simulink model "F16ASYM_Controlled"  (R2015a)
settings: Solver=ode3  SolverMode=SingleTasking  StartTime=0.0  StopTime=inf  FixedStep=T_sim  RelTol=1e-3
InitFcn:
  | load('NN_c_weights_Last_stable.mat')
StopFcn:
  | Final_results
values from neighbouring files (symbols this model uses):
  a1 = fitresult.p1    [Stall_protection.m]
  alpha_map_eval = ones(size(M_eval))*NaN    [Auto_trim_aid.m]    (also in Autotrim_maps.mat = [nan nan 0.277598136245 0.119432432992 0.0579479097061 0.027)
  beta_map_eval = ones(size(M_eval))*NaN    [Auto_trim_aid.m]    (also in Autotrim_maps.mat = [nan nan -0.00151549403324 0.00117807579006 -0.0052086799721)
  C_L_0 = fitresult.p2    [Stall_protection.m]
  G_eval = NaN*ones(size(M_sq,2),size(H_sq,2))    [Stall_protection.m]
  H_sq = unique(sort(H_sq))    [Stall_protection.m]
  H_sq_autotrim = min( F_envelope.H_1g):2000:max(F_envelope.H_1g)    [Auto_trim_aid.m]    (also in Autotrim_maps.mat = [0 2000 4000 6000 8000 10000 12000 14000 16000 18000])
  K_b_q_extrap_ACC = K_b_q_extrap    [RUN_ME.m]
  K_b_q_extrap_AoA = K_b_q_extrap    [RUN_ME.m]
  M_sq = unique(sort(M_sq))    [Stall_protection.m]
  M_sq_autotrim = 0:0.1:max(F_envelope.M_1g)    [Auto_trim_aid.m]    (also in Autotrim_maps.mat = [0 0.1 0.2 0.3 0.4 0.5 0.6 0.7 0.8 0.9 1 1.1 ... (21 element)
  T_sim = 0.02    [RUN_ME.m]
  tau_q_extrap_ACC = tau_q_extrap    [RUN_ME.m]
  tau_q_extrap_AoA = tau_q_extrap    [RUN_ME.m]
  velocity = M_eval(I,J)*a    [Auto_trim_aid.m]
undefined symbols (not defined in the file or in its folder): ACCEL, B, Earth, fi_flag_Simulink, GYRO, H_sq_sche, k_B, K_b_ACC_extrap, K_b_AoA_extrap, latitude, longitude, m, m_B, M_sq_sche, Model_used_flag, rad, s, sigbuilder_block, Stall_curve, tau_ACC_extrap, tau_AoA_extrap, Theta_1_roll_last, Theta_2_roll_last, Theta_3_roll_last, trim_control, trim_state, trim_throttle, V_Comp_A_w_z_last, V_Comp_last, V_Comp_last_ONE, V_long_lastA_w_z, V_long_lastAoA, V_roll_last, V_roll_lastMOD, V_yaw_last, W_Comp_A_w_z_last, W_Comp_last, W_long_lastA_w_z, W_long_lastAoA, W_roll_last, W_roll_lastMOD, W_yaw_last, WGS84
libraries: Adaptive_FaultTolerantControl x57, dspsigops x37, F16_Actuator_Library x14, commnoisgen2 x13, simulink x11, simulink_extras x10, dsparch4 x6, aerolibatmos2 x6, aerolibtransform2 x6, aerolibfltsims x3, dspvision x3, dspsnks4 x3
(part 12 of 14)

== system F16ASYM_Controlled/Primary Controller/P controller + adaptive Isolated NN/On-line (adaptive) multi-layer NNs SIMPL/Roll NN/Roll 2HL NN ==
  note: Be careful with dimensions of inputs!!!
      | NORMALIZATION!!!
  v_ad^ prev : Inport
  p_chanel vars : Inport  Port=2
  All_meas : Inport  Port=3
  Roll_learning rate : Inport  Port=4
  Roll reg param : Inport  Port=5
  " " : ToWorkspace  VariableName=Theta_3_roll_last  SampleTime=-1
      settings: MaxDataPoints=1
  "  " : Memory  X0=Theta_3_roll_last
  "   " : Memory  X0=Theta_2_roll_last
  B : Constant
  Bus Selector1 : BusSelector  OutputSignals=p_err,p_sf,p_sf_dot,K_b_p
  Bus Selector2 : BusSelector  OutputSignals=signal1.Alt meas (m),signal2.Mach,signal1.AoA meas (rad),signal1.SS meas (rad),signal1.omega_b meas (rad/s)
  Constant : Constant
  Constant2 : Constant
  Display : Display
  Divide : Product  Inputs=**
  Divide1 : Product  Inputs=**
  Divide2 : Product  Inputs=*/
  Gain : Gain  Gain=1/15000
  Memory2 : Memory  X0=Theta_1_roll_last
  Mux : Mux  Inputs=12
  Roll Multilayer NN : MATLAB Function  TreatAsAtomicUnit=on
  Scope : Scope
      settings: YMin=-14  YMax=4  SaveName=ScopeData16
  Selector : Selector  InputPortWidth=3  Indices=3
  Terminator : Terminator
  Terminator1 : Terminator
  To Workspace : ToWorkspace  VariableName=Theta_1_roll_last  SampleTime=-1
      settings: MaxDataPoints=1
  To Workspace1 : ToWorkspace  VariableName=Theta_2_roll_last  SampleTime=-1
      settings: MaxDataPoints=1
  v_ad_comp : Outport
  wires:
  Roll Multilayer NN/3(Z_norm_unit) -> Terminator1/1
  Mux/1 -> Roll Multilayer NN/1(X_bar), Scope/1, Display/1
  Roll reg param/1 -> Roll Multilayer NN/6(Roll_reg_param)
  Roll_learning rate/1 -> Roll Multilayer NN/5(Roll_learnign_rate)
  Memory2/1 -> Roll Multilayer NN/7(Theta_1)
  Roll Multilayer NN/5(Theta_2_update) -> "   "/1, To Workspace1/1
  "  "/1 -> Roll Multilayer NN/9(Theta_3)
  Roll Multilayer NN/6(Theta_3_update) -> " "/1, "  "/1
  Bus Selector2/2 -> Mux/3, Divide/1, Divide/2  "<Mach>"
  Constant2/1 -> Divide2/1
  Bus Selector1/4 -> Divide2/2  "<K_b_p>"
  Divide2/1 -> [P]
  Roll Multilayer NN/2(v_ad) -> Terminator/1
  Roll Multilayer NN/4(Theta_1_update) -> Memory2/1, To Workspace/1
  v_ad^ prev/1 -> Mux/12
  [P] -> Roll Multilayer NN/3(P)
  B/1 -> Roll Multilayer NN/4(B)
  "   "/1 -> Roll Multilayer NN/8(Theta_2)
  Roll Multilayer NN/1(v_ad_comp) -> v_ad_comp/1
  Selector/1 -> Mux/8
  Bus Selector2/5 -> Selector/1  "<omega_b meas (rad/s)>"
  Gain/1 -> Mux/2
  Bus Selector2/4 -> Mux/7  "<SS meas (rad)>"
  Divide1/1 -> Mux/6
  Bus Selector2/3 -> Mux/5, Divide1/1, Divide1/2  "<AoA meas (rad)>"
  Divide/1 -> Mux/4
  Bus Selector2/1 -> Gain/1  "<Alt meas (m)>"
  All_meas/1 -> Bus Selector2/1
  Constant/1 -> Mux/1
  Bus Selector1/1 -> Roll Multilayer NN/2(e), Mux/9  "<p_err>"
  Bus Selector1/3 -> Mux/11  "<p_sf_dot>"
  Bus Selector1/2 -> Mux/10  "<p_sf>"
  p_chanel vars/1 -> Bus Selector1/1

== system F16ASYM_Controlled/Primary Controller/P controller + adaptive Isolated NN/On-line (adaptive) multi-layer NNs SIMPL/Yaw Chanel/Yaw HL NN ==
  note: Be careful with dimensions of inputs!!!
      | NORMALIZATION!!!
  v_ad^ prev : Inport
  Yaw_chanel vars : Inport  Port=2
  All_meas : Inport  Port=3
  Yaw_learning rate : Inport  Port=4
  Yaw reg param : Inport  Port=5
  Bus Selector1 : BusSelector  OutputSignals=beta_chanel vars.beta_err,r_chanel vars.r_err,beta_chanel vars.beta_sf,beta_chanel vars.beta_sf_dot,r_chanel vars.r_sf_dot,beta_chanel vars.K_b_beta,r_chanel vars.K_b_r
  Bus Selector2 : BusSelector  OutputSignals=signal1.Alt meas (m),signal2.Mach,signal1.AoA meas (rad),signal1.Euler meas (rad)
  Constant : Constant
  Constant1 : Constant  Value=[0;1]
  Display : Display
  Divide : Product  Inputs=**
  Gain : Gain  Gain=1/15000
  Memory2 : Memory  X0=V_yaw_last
  Memory3 : Memory  X0=W_yaw_last
  Mux : Mux  Inputs=12
  Mux1 : Mux  Inputs=2
  Mux2 : Mux  Inputs=2
  Scope : Scope
      settings: YMin=-0.25  YMax=3.75  SaveName=ScopeData17
  Selector : Selector  InputPortWidth=3
  Terminator : Terminator
  Terminator1 : Terminator
  To Workspace : ToWorkspace  VariableName=V_yaw_last  SampleTime=-1
      settings: MaxDataPoints=1
  To Workspace1 : ToWorkspace  VariableName=W_yaw_last  SampleTime=-1
      settings: MaxDataPoints=1
  Yaw NN : MATLAB Function  TreatAsAtomicUnit=on
  v_ad_comp : Outport
  wires:
  Yaw NN/3(Z_norm_unit) -> Terminator1/1
  Mux/1 -> Yaw NN/1(X_bar), Scope/1, Display/1
  Bus Selector1/3 -> Mux/9  "<beta_sf>"
  Bus Selector1/1 -> Mux/7, Mux1/1  "<beta_err>"
  Bus Selector1/4 -> Mux/10  "<beta_sf_dot>"
  Bus Selector1/2 -> Mux/8, Mux1/2  "<r_err>"
  Bus Selector1/5 -> Mux/11  "<r_sf_dot>"
  Selector/1 -> Mux/6
  Bus Selector2/3 -> Mux/5  "<AoA meas (rad)>"
  Bus Selector2/2 -> Mux/3, Divide/1, Divide/2  "<Mach>"
  Gain/1 -> Mux/2
  Bus Selector2/4 -> Selector/1  "<Euler meas (rad)>"
  Yaw NN/2(v_ad) -> Terminator/1
  Yaw NN/5(V_update) -> To Workspace/1, Memory2/1
  v_ad^ prev/1 -> Mux/12
  [Ks] -> Yaw NN/3(Ks)
  Constant1/1 -> Yaw NN/4(B)
  Memory3/1 -> Yaw NN/7(W)
  Memory2/1 -> Yaw NN/8(V)
  Yaw NN/4(W_update) -> To Workspace1/1, Memory3/1
  Yaw NN/1(v_ad_comp) -> v_ad_comp/1
  Yaw_chanel vars/1 -> Bus Selector1/1
  Yaw_learning rate/1 -> Yaw NN/5(Long_learnign_rate)
  Yaw reg param/1 -> Yaw NN/6(Long_reg_param)
  Constant/1 -> Mux/1
  All_meas/1 -> Bus Selector2/1
  Bus Selector2/1 -> Gain/1  "<Alt meas (m)>"
  Divide/1 -> Mux/4
  Mux1/1 -> Yaw NN/2(e)  "e"
  Bus Selector1/7 -> Mux2/2  "<K_b_r>"
  Bus Selector1/6 -> Mux2/1  "<K_b_beta>"
  Mux2/1 -> [Ks]

== system F16ASYM_Controlled/Primary Controller/PI Primary Controller/Longitudinal Controller: AoA or A_w_z/Longitudinal controller in A_w_z/Accel rate --> AoA rate! ==
  A_w_z dot : Inport
  All_meas : Inport  Port=2
  1/a_1 : Gain  Gain=1/a1
  Bus Selector : BusSelector  OutputSignals=signal2.q (Pa)
  Divide : Product  Inputs=**
  Divide1 : Product  Inputs=**
  Divide2 : Product  Inputs=*/
  S : Constant  Value=27.87
  mass : Constant  Value=9295.44
  alpha_dot des : Outport
  wires:
  1/a_1/1 -> alpha_dot des/1  "ALPHA_DOT"
  All_meas/1 -> Bus Selector/1
  Divide2/1 -> 1/a_1/1
  Divide/1 -> Divide2/2
  Divide1/1 -> Divide2/1
  mass/1 -> Divide1/2
  Bus Selector/1 -> Divide/2  "<q (Pa)>"
  S/1 -> Divide/1
  A_w_z dot/1 -> Divide1/1

== system F16ASYM_Controlled/SI and FDI/SI and FDI: Realistic/FDI: Assumed?/Delays/1st order model ==
  y_in : Inport
  y_initial : Inport  Port=2
  Enable : EnablePort  StatesWhenEnabling=reset
  Add : Sum  Inputs=|+-
  Integrator : Integrator  InitialConditionSource=external  InitialCondition=y_i
  K_ref : Gain  Gain=K_ref
  y_out : Outport
  wires:
  Integrator/1 -> Add/2, y_out/1
  K_ref/1 -> Integrator/1
  Add/1 -> K_ref/1
  y_in/1 -> Add/1
  y_initial/1 -> Integrator/2

== system F16ASYM_Controlled/SI and FDI/SI and FDI: Realistic/FDI: Assumed?/Delays/1st order model1 ==
  y_in : Inport
  y_initial : Inport  Port=2
  Enable : EnablePort  StatesWhenEnabling=reset
  Add : Sum  Inputs=|+-
  Integrator : Integrator  InitialConditionSource=external  InitialCondition=y_i
  K_ref : Gain  Gain=K_ref
  y_out : Outport
  wires:
  y_initial/1 -> Integrator/2
  y_in/1 -> Add/1
  Add/1 -> K_ref/1
  K_ref/1 -> Integrator/1
  Integrator/1 -> y_out/1, Add/2

== system F16ASYM_Controlled/SI and FDI/SI and FDI: Realistic/FDI: Assumed?/Delays/1st order model2 ==
  y_in : Inport
  y_initial : Inport  Port=2
  Enable : EnablePort  StatesWhenEnabling=reset
  Add : Sum  Inputs=|+-
  Integrator : Integrator  InitialConditionSource=external  InitialCondition=y_i
  K_ref : Gain  Gain=K_ref
  y_out : Outport
  wires:
  y_initial/1 -> Integrator/2
  y_in/1 -> Add/1
  Add/1 -> K_ref/1
  K_ref/1 -> Integrator/1
  Integrator/1 -> y_out/1, Add/2

== system F16ASYM_Controlled/SI and FDI/SI and FDI: Realistic/FDI: Assumed?/Delays/1st order model3 ==
  y_in : Inport
  y_initial : Inport  Port=2
  Enable : EnablePort  StatesWhenEnabling=reset
  Add : Sum  Inputs=|+-
  Integrator : Integrator  InitialConditionSource=external  InitialCondition=y_i
  K_ref : Gain  Gain=K_ref
  y_out : Outport
  wires:
  y_initial/1 -> Integrator/2
  y_in/1 -> Add/1
  Add/1 -> K_ref/1
  K_ref/1 -> Integrator/1
  Integrator/1 -> y_out/1, Add/2

== system F16ASYM_Controlled/SI and FDI/SI and FDI: Realistic/FDI: Assumed?/Delays/1st order model4 ==
  y_in : Inport
  y_initial : Inport  Port=2
  Enable : EnablePort  StatesWhenEnabling=reset
  Add : Sum  Inputs=|+-
  Integrator : Integrator  InitialConditionSource=external  InitialCondition=y_i
  K_ref : Gain  Gain=K_ref
  y_out : Outport
  wires:
  y_initial/1 -> Integrator/2
  y_in/1 -> Add/1
  Add/1 -> K_ref/1
  K_ref/1 -> Integrator/1
  Integrator/1 -> y_out/1, Add/2

== system F16ASYM_Controlled/SI and FDI/SI and FDI: Realistic/FDI: Assumed?/Delays/1st order model5 ==
  y_in : Inport
  y_initial : Inport  Port=2
  Enable : EnablePort  StatesWhenEnabling=reset
  Add : Sum  Inputs=|+-
  Integrator : Integrator  InitialConditionSource=external  InitialCondition=y_i
  K_ref : Gain  Gain=K_ref
  y_out : Outport
  wires:
  y_initial/1 -> Integrator/2
  y_in/1 -> Add/1
  Add/1 -> K_ref/1
  K_ref/1 -> Integrator/1
  Integrator/1 -> y_out/1, Add/2

== system F16ASYM_Controlled/SI and FDI/SI and FDI: Realistic/FDI: Assumed?/Delays/1st order model6 ==
  y_in : Inport
  y_initial : Inport  Port=2
  Enable : EnablePort  StatesWhenEnabling=reset
  Add : Sum  Inputs=|+-
  Integrator : Integrator  InitialConditionSource=external  InitialCondition=y_i
  K_ref : Gain  Gain=K_ref
  y_out : Outport
  wires:
  y_initial/1 -> Integrator/2
  y_in/1 -> Add/1
  Add/1 -> K_ref/1
  K_ref/1 -> Integrator/1
  Integrator/1 -> y_out/1, Add/2

== system F16ASYM_Controlled/Primary Controller/P con  + Crossed NN + AWU+Lim + hand-over+Scheduling/P controller + adaptive Crossed NN + AWU+Lim    in ACC /Body Rates Controller/Ref Model and P Controller1/Reference Model ==
  y_ref : Inport
  tau : Inport  Port=2
  Add : Sum  Inputs=|+-
  Constant : Constant
  Integrator : Integrator  InitialCondition=trim_state(11)
  "K_ref " : Product  Inputs=*/
  K_ref prod : Product  Inputs=**
  y_c_dot : Outport
  y_c : Outport  Port=2
  wires:
  y_ref/1 -> Add/1
  Add/1 -> K_ref prod/1
  K_ref prod/1 -> Integrator/1, y_c_dot/1
  Integrator/1 -> y_c/1, Add/2
  tau/1 -> "K_ref "/2
  Constant/1 -> "K_ref "/1
  "K_ref "/1 -> K_ref prod/2

== system F16ASYM_Controlled/Primary Controller/P con  + Crossed NN + AWU+Lim + hand-over+Scheduling/P controller + adaptive Crossed NN + AWU+Lim    in ACC /Longitudinal controller in A_w_z/Ref Model and P Controller1/Reference Model ==
  y_ref : Inport
  tau : Inport  Port=2
  Add : Sum  Inputs=|+-
  Constant : Constant
  Integrator : Integrator
  "K_ref " : Product  Inputs=*/
  K_ref prod : Product  Inputs=**
  y_c_dot : Outport
  y_c : Outport  Port=2
  wires:
  y_ref/1 -> Add/1
  Add/1 -> K_ref prod/1
  K_ref prod/1 -> Integrator/1, y_c_dot/1
  Integrator/1 -> y_c/1, Add/2
  tau/1 -> "K_ref "/2
  Constant/1 -> "K_ref "/1
  "K_ref "/1 -> K_ref prod/2

== system F16ASYM_Controlled/Primary Controller/P con  + Crossed NN + AWU+Lim + hand-over+Scheduling/P controller + adaptive Crossed NN + AWU+Lim   in AoA/Body Rates Controller/Ref Model and P Controller1/Reference Model ==
  y_ref : Inport
  tau : Inport  Port=2
  Add : Sum  Inputs=|+-
  Constant : Constant
  Integrator : Integrator  InitialCondition=trim_state(11)
  "K_ref " : Product  Inputs=*/
  K_ref prod : Product  Inputs=**
  y_c_dot : Outport
  y_c : Outport  Port=2
  wires:
  y_ref/1 -> Add/1
  Add/1 -> K_ref prod/1
  K_ref prod/1 -> Integrator/1, y_c_dot/1
  Integrator/1 -> y_c/1, Add/2
  tau/1 -> "K_ref "/2
  Constant/1 -> "K_ref "/1
  "K_ref "/1 -> K_ref prod/2

== system F16ASYM_Controlled/Primary Controller/P con  + Crossed NN + AWU+Lim + hand-over+Scheduling/P controller + adaptive Crossed NN + AWU+Lim   in AoA/Longitudinal controller in AoA1/Ref Model and P Controller1/Reference Model ==
  y_ref : Inport
  tau : Inport  Port=2
  Add : Sum  Inputs=|+-
  Constant : Constant
  Integrator : Integrator  InitialCondition=trim_state(8)
  "K_ref " : Product  Inputs=*/
  K_ref prod : Product  Inputs=**
  y_c_dot : Outport
  y_c : Outport  Port=2
  wires:
  y_ref/1 -> Add/1
  Add/1 -> K_ref prod/1
  K_ref prod/1 -> Integrator/1, y_c_dot/1
  Integrator/1 -> y_c/1, Add/2
  tau/1 -> "K_ref "/2
  Constant/1 -> "K_ref "/1
  "K_ref "/1 -> K_ref prod/2

== system F16ASYM_Controlled/Primary Controller/P con + adaptive Crossed NN + AWU+Lim + Scheduling/Body Rates Controller/Body Rates Controller  in ACC/Ref Model and P Controller1/Reference Model ==
  y_ref : Inport
  tau : Inport  Port=2
  Add : Sum  Inputs=|+-
  Constant : Constant
  Integrator : Integrator  InitialCondition=trim_state(11)
  "K_ref " : Product  Inputs=*/
  K_ref prod : Product  Inputs=**
  y_c_dot : Outport
  y_c : Outport  Port=2
  wires:
  y_ref/1 -> Add/1
  Add/1 -> K_ref prod/1
  K_ref prod/1 -> Integrator/1, y_c_dot/1
  Integrator/1 -> y_c/1, Add/2
  tau/1 -> "K_ref "/2
  Constant/1 -> "K_ref "/1
  "K_ref "/1 -> K_ref prod/2

== system F16ASYM_Controlled/Primary Controller/P con + adaptive Crossed NN + AWU+Lim + Scheduling/Body Rates Controller/Body Rates Controller in  AoA/Ref Model and P Controller1/Reference Model ==
  y_ref : Inport
  tau : Inport  Port=2
  Add : Sum  Inputs=|+-
  Constant : Constant
  Integrator : Integrator  InitialCondition=trim_state(11)
  "K_ref " : Product  Inputs=*/
  K_ref prod : Product  Inputs=**
  y_c_dot : Outport
  y_c : Outport  Port=2
  wires:
  y_ref/1 -> Add/1
  Add/1 -> K_ref prod/1
  K_ref prod/1 -> Integrator/1, y_c_dot/1
  Integrator/1 -> y_c/1, Add/2
  tau/1 -> "K_ref "/2
  Constant/1 -> "K_ref "/1
  "K_ref "/1 -> K_ref prod/2

== system F16ASYM_Controlled/Primary Controller/P con + adaptive Crossed NN + AWU+Lim + Scheduling/Longitudinal Controller: AoA or A_w_z/Longitudinal controller in A_w_z/Ref Model and P Controller1/Reference Model ==
  y_ref : Inport
  tau : Inport  Port=2
  Add : Sum  Inputs=|+-
  Constant : Constant
  Integrator : Integrator
  "K_ref " : Product  Inputs=*/
  K_ref prod : Product  Inputs=**
  y_c_dot : Outport
  y_c : Outport  Port=2
  wires:
  y_ref/1 -> Add/1
  Add/1 -> K_ref prod/1
  K_ref prod/1 -> Integrator/1, y_c_dot/1
  Integrator/1 -> y_c/1, Add/2
  tau/1 -> "K_ref "/2
  Constant/1 -> "K_ref "/1
  "K_ref "/1 -> K_ref prod/2

== system F16ASYM_Controlled/Primary Controller/P con + adaptive Crossed NN + AWU+Lim + Scheduling/Longitudinal Controller: AoA or A_w_z/Longitudinal controller in AoA/Ref Model and P Controller1/Reference Model ==
  y_ref : Inport
  tau : Inport  Port=2
  Add : Sum  Inputs=|+-
  Constant : Constant
  Integrator : Integrator  InitialCondition=trim_state(8)
  "K_ref " : Product  Inputs=*/
  K_ref prod : Product  Inputs=**
  y_c_dot : Outport
  y_c : Outport  Port=2
  wires:
  y_ref/1 -> Add/1
  Add/1 -> K_ref prod/1
  K_ref prod/1 -> Integrator/1, y_c_dot/1
  Integrator/1 -> y_c/1, Add/2
  tau/1 -> "K_ref "/2
  Constant/1 -> "K_ref "/1
  "K_ref "/1 -> K_ref prod/2

== matlab function F16ASYM_Controlled/Primary Controller/P controller + adaptive Isolated NN/On-line (adaptive) multi-layer NNs/Roll NN/Roll 2HL NN/Roll Multilayer NN ==
  data: X_bar input size=[12,1]; v_ad_comp output; e input size=1; P input; B input; Roll_learnign_rate input size=1; Roll_reg_param input size=1; Theta_1 input size=[30,12]; Theta_2 input size=[20,31]; Theta_3 input size=[1,21]; v_ad output; Z_norm_unit output; T_sim parameter; Theta_1_update output; Theta_2_update output; Theta_3_update output
function [v_ad_comp,v_ad,Z_norm_unit,Theta_1_update,Theta_2_update,Theta_3_update]  = Roll_ML_NN(X_bar,e,P,B,Roll_learnign_rate, Roll_reg_param,Theta_1,Theta_2,Theta_3,T_sim)

%% Compute prelimiary parameters
zeta= e'*P*B;

%% Feedforward. Layers: Sigmoidal, linear, linear

a2=[1 ;  sigmoid( Theta_1*X_bar )]; % Sigmoidal
a3=[1 ;  (Theta_2*a2)]; % Linear
% z4=Theta_3*a3;
% a4 = z4; % Linear
% v_ad =a4;

% Backward
% % delta4=zeta; % In this particular case of adaptive NN, this error is a weighted tracking error
delta3=Theta_3'*zeta;
delta2=Theta_2'*delta3(2:end).*(a2.*(ones(size(a2))-a2)); 


%% Compute the gradients or adaptation laws
Gamma_Theta_3= Roll_learnign_rate; %  learnign rate
Gamma_Theta_2 = Roll_learnign_rate; % learning rate
Gamma_Theta_1= Roll_learnign_rate; % learning rate
lambda = Roll_reg_param;    % Regularization constant

% % Theta_1_dot=zeros(size(Theta_1));
% % Theta_2_dot=zeros(size(Theta_2));
% % Theta_3_dot=zeros(size(Theta_3));

Theta_3_dot = -Gamma_Theta_3*zeta*a3' ;
Theta_3_dot(:,2:end) =  Theta_3_dot(:,2:end) - Gamma_Theta_3*lambda*norm(zeta).*Theta_3(:,2:end);

Theta_2_dot= -Gamma_Theta_2*( delta3(2:end)*a2'   + lambda*norm(zeta).*Theta_2);
Theta_2_dot(:,2:end) =  Theta_2_dot(:,2:end) - Gamma_Theta_2*lambda*norm(zeta).*Theta_2(:,2:end);

Theta_1_dot= -Gamma_Theta_1*( delta2(2:end)*X_bar'   + lambda*norm(zeta).*Theta_1);
Theta_1_dot(:,2:end) =  Theta_1_dot(:,2:end) - Gamma_Theta_1*lambda*norm(zeta).*Theta_1(:,2:end);


%% Adaptation
Theta_1_update = Theta_1 + T_sim*Theta_1_dot;
Theta_2_update = Theta_2 + T_sim*Theta_2_dot;
Theta_3_update = Theta_3 + T_sim*Theta_3_dot;

%% re-compute v_ad

a2=[1 ;  sigmoid( Theta_1_update*X_bar )]; % Sigmoidal
a3=[1 ;  (Theta_2_update*a2)]; % Linear
v_ad=Theta_3_update*a3;


%% Compute v_ad_comp
% Z = blkdiag( Theta_1_update , Theta_2_update , Theta_3_update );

Z =  [ Theta_1_update, zeros(size(Theta_1_update,1),size(Theta_2_update,2)) , zeros(size(Theta_1_update,1),size(Theta_3_update,2));
            zeros(size(Theta_2_update,1),size(Theta_1_update,2)) , Theta_2_update , zeros(size(Theta_2_update,1),size(Theta_3_update,2)) ;
            zeros(size(Theta_3_update,1),size(Theta_1_update,2)),zeros(size(Theta_3_update,1),size(Theta_2_update,2)),  Theta_3_update ];

Z_norm = norm(Z,'fro');
Z_max = min(size(Theta_1))*min(size(Theta_2))*min(size(Theta_3));
Z_norm_unit = Z_norm;

K_r0= 0.02;
K_r1= 0;
v_r0 = -K_r0*zeta;
v_r1 = -K_r1*(Z_norm+Z_max)*zeta;

v_ad_comp = v_ad + v_r1 +v_r0;


end

== matlab function F16ASYM_Controlled/Faults injection/MATLAB Function ==
  data: reconfig_params output; Delta_mass input; Delta_S_L input; Delta_S_R input; Delta_S_Fin input; xcg input; Delta_J input; Eff input; Deltas_coef input
function reconfig_params  = Reconfig_params(Delta_mass,Delta_S_L,Delta_S_R,Delta_S_Fin,xcg,Delta_J,Eff,Deltas_coef)

reconfig_params= zeros(19,1);

S_L  = 27.87/2;
S_R = 27.87/2;
S_fin = 6.578;

if size(Eff,2)==7
    Eff=Eff';
end
if size(Deltas_coef,2)==3
    Deltas_coef=Deltas_coef';
end

reconfig_params(1)= 9295.44*(1+Delta_mass); % mass
reconfig_params(2) = S_L*0.3 + 0.7*S_L*(1-Delta_S_L); % S_current_L. Split between 0.2 and 0.8 because it would imposible to lose a 100% which is part of fuselage 
reconfig_params(3) = S_R*0.3 + 0.7*S_R*(1-Delta_S_R); % S_current_R
reconfig_params(4) = S_fin*0.1 + 0.9*S_fin*(1-Delta_S_Fin);   % S_fin_current
reconfig_params(5) = xcg;  % xcg
reconfig_params(6) = 75673.6*(1+Delta_J(1)); % Jy
reconfig_params(7) = 1331.4*(1+Delta_J(2));  % Jxz
reconfig_params(8)  = 85552.1*(1+Delta_J(3)); % Jz
reconfig_params(9) = 12874.8*(1+Delta_J(4));   % Jx
reconfig_params(10:16)  = Eff; % Effectiveness
reconfig_params(17:19)  = Deltas_coef; %Deltas lift, drag and pitching moment

end

== matlab function F16ASYM_Controlled/Primary Controller/P controller + adaptive Isolated NN/On-line (adaptive) multi-layer NNs/Roll NN/Roll 1HL NN/Roll NN ==
  data: X_bar input size=[12,1]; v_ad_comp output; e input; P input; B input; Roll_learnign_rate input size=1; Roll_reg_param input size=1; W input size=[1,31]; V input size=[30,12]; v_ad output; Z_norm_unit output; T_sim parameter; W_update output size=[1,31]; V_update output size=[30,12]
function [v_ad_comp,v_ad,Z_norm_unit,W_update,V_update]  = Roll_NN(X_bar,e,P,B,Roll_learnign_rate,Roll_reg_param,W,V,T_sim)

%% Compute prelimiary parametes
zeta= e'*P*B;
s=zeros(30,1);
z=s;
%% Feedforward
z = V*X_bar;
s=sigmoid(V*X_bar);

sigma = [1 ; s ];
% v_ad = W*sigma;

sigma_grad = (sigma.*(ones(size(sigma))-sigma));

%% Compute the gradients or adaptation laws
Gamma_w= Roll_learnign_rate; % W learnign rate
Gamma_v= Roll_learnign_rate; %V learning rate
lambda = Roll_reg_param;

V_dot=zeros(size(V));
W_dot=zeros(size(W'));

W_dot= -Gamma_w*(  (sigma - sigma_grad.*[1;z] ).*zeta  );
W_dot(2:end,1)= W_dot(2:end,1) - Gamma_w*lambda*norm(zeta)*(W(:,2:end))';

M = W'*zeta.*sigma_grad ;
V_dot= -Gamma_v*( M(2:end)*X_bar'  );
V_dot(:,2:end)= V_dot(:,2:end) - Gamma_v*lambda*norm(zeta).*V(:,2:end);


% Other way: Based on notes of Andrew NG
% % % W_dot=zeros(size(W));
% % % delta2=W'*zeta.*sigma_grad;
% % % 
% % % V_dot = - Gamma_v*( delta2(2:end)*X_bar');
% % % V_dot(:,2:end)= V_dot(:,2:end) - Gamma_v*lambda*norm(zeta).*V(:,2:end);
% % % 
% % % W_dot = - Gamma_w*( zeta*sigma');
% % % W_dot(:,2:end)= W_dot(:,2:end) - Gamma_w*lambda*norm(zeta)*(W(:,2:end));
% % % 
% % % W_dot = W_dot';


%% Adaptation
W_update = W + T_sim*W_dot';
V_update = V + T_sim*V_dot;

%% re-compute v_ad

z = V*X_bar;
s=sigmoid(V*X_bar);

sigma = [1 ; s(:,1) ];
v_ad = W*sigma;

%% Compute v_ad_comp
Z = [ V,zeros(size(V,1),size(W,2));
    zeros(size(W,1),size(V,2)),W];
    
Z_norm = norm(Z,'fro');
Z_max = 2*min(size(W,1),size(W,2) )*min( size(V,1),size(V,2) );
Z_norm_unit = Z_norm;

K_r0= 0;
K_r1= 0;
v_r0 = -K_r0*zeta;
v_r1 = -K_r1*(Z_norm+Z_max)*zeta;
v_ad_comp = v_ad + v_r1 +v_r0;

% % K_r1= 1;
% % v_r1 = - K_r1*(Z_norm+Z_max)*zeta;
% % 
% % v_ad_comp = v_ad + v_r1 ;



end

== matlab function F16ASYM_Controlled/Primary Controller/P controller + adaptive Isolated NN/On-line (adaptive) multi-layer NNs/Long Chanel/Long HL NN AoA/Long NN ==
  data: X_bar input size=[10,1]; v_ad_comp output; e input; Ks input; B input; Long_learnign_rate input size=1; Long_reg_param input size=1; W input size=[1,31]; V input size=[30,10]; v_ad output; Z_norm_unit output; T_sim parameter; W_update output; V_update output
function [v_ad_comp,v_ad,Z_norm_unit,W_update,V_update]  = Long_AoA_NN(X_bar,e, Ks,B,Long_learnign_rate,Long_reg_param,W,V,T_sim)

%% Compute prelimiary parametes Ks(1)=K_b_alpha  and Ks(2) = K_b_q
P = [   1/Ks(1) , 1/(Ks(1)^2+Ks(1)*Ks(2));
     1/(Ks(1)^2+Ks(1)*Ks(2)) ,(Ks(1)^2+Ks(1)*Ks(2)+1)/(Ks(2)^2*Ks(1)+Ks(2)*Ks(1)^2) ];
zeta= e'*P*B;
s=zeros(30,1);
z=s;
%% Feedforward
z = V*X_bar;
s=sigmoid(V*X_bar);

sigma = [1 ; s ];
% v_ad = W*sigma;

sigma_grad = (sigma.*(ones(size(sigma))-sigma));

%% Compute the gradients or adaptation laws
Gamma_w= Long_learnign_rate; % W learnign rate
Gamma_v= Long_learnign_rate; %V learning rate
lambda = Long_reg_param;

V_dot=zeros(size(V));
W_dot=zeros(size(W'));

W_dot= -Gamma_w*(  (sigma - sigma_grad.*[1;z] ).*zeta  );
W_dot(2:end,1)= W_dot(2:end,1) - Gamma_w*lambda*norm(zeta)*(W(:,2:end))';

M = W'*zeta.*sigma_grad ;
V_dot= -Gamma_v*( M(2:end)*X_bar'  );
V_dot(:,2:end)= V_dot(:,2:end) - Gamma_v*lambda*norm(zeta).*V(:,2:end);


% % % Other way: Based on notes of Andrew NG
% % W_dot=zeros(size(W));
% % delta2=W'*zeta.*sigma_grad;
% % 
% % V_dot = - Gamma_v*( delta2(2:end)*X_bar');
% % V_dot(:,2:end)= V_dot(:,2:end) - Gamma_v*lambda*norm(zeta).*V(:,2:end);
% % 
% % W_dot = - Gamma_w*( zeta*sigma');
% % W_dot(:,2:end)= W_dot(:,2:end) - Gamma_w*lambda*norm(zeta)*(W(:,2:end));
% % 
% % W_dot = W_dot';


%% Adaptation
W_update = W + T_sim*W_dot';
V_update = V + T_sim*V_dot;

%% re-compute v_ad

z = V*X_bar;
s=sigmoid(V*X_bar);

sigma = [1 ; s(:,1) ];
v_ad = W*sigma;

%% Compute v_ad_comp
Z = [ V,zeros(size(V,1),size(W,2));
    zeros(size(W,1),size(V,2)),W];
    
Z_norm = norm(Z,'fro');
Z_max = 2*min(size(W,1),size(W,2) )*min( size(V,1),size(V,2) );
Z_norm_unit = Z_norm;

K_r0= 0.02;
K_r1= 0;
v_r0 = -K_r0*zeta;
v_r1 = -K_r1*(Z_norm+Z_max)*zeta;

v_ad_comp = v_ad + v_r1 +v_r0;


end

== matlab function F16ASYM_Controlled/Primary Controller/P controller + adaptive Isolated NN/On-line (adaptive) multi-layer NNs/Long Chanel/Long HL NN A_w_z/Long NN ==
  data: X_bar input size=[10,1]; v_ad_comp output; e input; F input; Ks input; B input; Long_learnign_rate input size=1; Long_reg_param input size=1; W input size=[1,31]; V input size=[30,10]; v_ad output; Z_norm_unit output; T_sim parameter; W_update output; V_update output
function [v_ad_comp,v_ad,Z_norm_unit,W_update,V_update]  = Long_AoA_NN(X_bar,e, F, Ks,B,Long_learnign_rate,Long_reg_param,W,V,T_sim)

%% Compute prelimiary parametes Ks(1)=K_b_alpha  and Ks(2) = K_b_q
P = [   1/Ks(1) , F/(Ks(1)^2+Ks(1)*Ks(2));
     1/(Ks(1)^2+Ks(1)*Ks(2)) ,(Ks(1)^2+Ks(1)*Ks(2)+F^2)/(Ks(2)^2*Ks(1)+Ks(2)*Ks(1)^2) ];
zeta= e'*P*B;
s=zeros(30,1);
z=s;
%% Feedforward
z = V*X_bar;
s=sigmoid(V*X_bar);

sigma = [1 ; s ];
% v_ad = W*sigma;

sigma_grad = (sigma.*(ones(size(sigma))-sigma));

%% Compute the gradients or adaptation laws
Gamma_w= Long_learnign_rate; % W learnign rate
Gamma_v= Long_learnign_rate; %V learning rate
lambda = Long_reg_param;

V_dot=zeros(size(V));
W_dot=zeros(size(W'));

W_dot= -Gamma_w*(  (sigma - sigma_grad.*[1;z] ).*zeta  );
W_dot(2:end,1)= W_dot(2:end,1) - Gamma_w*lambda*norm(zeta)*(W(:,2:end))';

M = W'*zeta.*sigma_grad ;
V_dot= -Gamma_v*( M(2:end)*X_bar'  );
V_dot(:,2:end)= V_dot(:,2:end) - Gamma_v*lambda*norm(zeta).*V(:,2:end);


% % % Other way: Based on notes of Andrew NG
% % W_dot=zeros(size(W));
% % delta2=W'*zeta.*sigma_grad;
% % 
% % V_dot = - Gamma_v*( delta2(2:end)*X_bar');
% % V_dot(:,2:end)= V_dot(:,2:end) - Gamma_v*lambda*norm(zeta).*V(:,2:end);
% % 
% % W_dot = - Gamma_w*( zeta*sigma');
% % W_dot(:,2:end)= W_dot(:,2:end) - Gamma_w*lambda*norm(zeta)*(W(:,2:end));
% % 
% % W_dot = W_dot';


%% Adaptation
W_update = W + T_sim*W_dot';
V_update = V + T_sim*V_dot;

%% re-compute v_ad

z = V*X_bar;
s=sigmoid(V*X_bar);

sigma = [1 ; s(:,1) ];
v_ad = W*sigma;

%% Compute v_ad_comp
Z = [ V,zeros(size(V,1),size(W,2));
    zeros(size(W,1),size(V,2)),W];
    
Z_norm = norm(Z,'fro');
Z_max = 2*min(size(W,1),size(W,2) )*min( size(V,1),size(V,2) );
Z_norm_unit = Z_norm/Z_max;

K_r0= 0.1;
K_r1= 0.001;
v_r0 = -K_r0*zeta;
v_r1 = -K_r1*(Z_norm+Z_max)*zeta;

v_ad_comp = v_ad + v_r1 +v_r0;


end

== matlab function F16ASYM_Controlled/Primary Controller/P controller + adaptive Isolated NN/Sigmoid /MATLAB Function ==
  data: u input; y output; a input
function y = sigmoid_a(u,a)

y = 2.0 ./ (1.0 + exp(-a*u(1:3)))-1;

== matlab function F16ASYM_Controlled/Primary Controller/P controller + adaptive Isolated NN/On-line (adaptive) multi-layer NNs/Yaw Chanel/Yaw HL NN/Yaw NN ==
  data: X_bar input size=[12,1]; v_ad_comp output; e input; Ks input; B input; Long_learnign_rate input size=1; Long_reg_param input size=1; W input size=[1,31]; V input size=[30,12]; v_ad output; Z_norm_unit output; T_sim parameter; W_update output; V_update output
function [v_ad_comp,v_ad,Z_norm_unit,W_update,V_update]  = Yaw_NN(X_bar,e, Ks,B,Long_learnign_rate,Long_reg_param,W,V,T_sim)

%% Compute prelimiary parametes Ks(1)=K_b_alpha  and Ks(2) = K_b_q
P = [   1/Ks(1) , 1/(Ks(1)^2+Ks(1)*Ks(2));
     1/(Ks(1)^2+Ks(1)*Ks(2)) ,(Ks(1)^2+Ks(1)*Ks(2)+1)/(Ks(2)^2*Ks(1)+Ks(2)*Ks(1)^2) ];
zeta= e'*P*B;
s=zeros(30,1);
z=s;
%% Feedforward
z = V*X_bar;
s=sigmoid(V*X_bar);

sigma = [1 ; s ];
% v_ad = W*sigma;

sigma_grad = (sigma.*(ones(size(sigma))-sigma));

%% Compute the gradients or adaptation laws
Gamma_w= Long_learnign_rate; % W learnign rate
Gamma_v= Long_learnign_rate; %V learning rate
lambda = Long_reg_param;

V_dot=zeros(size(V));
W_dot=zeros(size(W'));

W_dot= -Gamma_w*(  (sigma - sigma_grad.*[1;z] ).*zeta  );
W_dot(2:end,1)= W_dot(2:end,1) - Gamma_w*lambda*norm(zeta)*(W(:,2:end))';

M = W'*zeta.*sigma_grad ;
V_dot= -Gamma_v*( M(2:end)*X_bar'  );
V_dot(:,2:end)= V_dot(:,2:end) - Gamma_v*lambda*norm(zeta).*V(:,2:end);


% % % Other way: Based on notes of Andrew NG
% % W_dot=zeros(size(W));
% % delta2=W'*zeta.*sigma_grad;
% % 
% % V_dot = - Gamma_v*( delta2(2:end)*X_bar');
% % V_dot(:,2:end)= V_dot(:,2:end) - Gamma_v*lambda*norm(zeta).*V(:,2:end);
% % 
% % W_dot = - Gamma_w*( zeta*sigma');
% % W_dot(:,2:end)= W_dot(:,2:end) - Gamma_w*lambda*norm(zeta)*(W(:,2:end));
% % 
% % W_dot = W_dot';


%% Adaptation
W_update = W + T_sim*W_dot';
V_update = V + T_sim*V_dot;

%% re-compute v_ad

z = V*X_bar;
s=sigmoid(V*X_bar);

sigma = [1 ; s(:,1) ];
v_ad = W*sigma;

%% Compute v_ad_comp
Z = [ V,zeros(size(V,1),size(W,2));
    zeros(size(W,1),size(V,2)),W];
    
Z_norm = norm(Z,'fro');
Z_max = 2*min(size(W,1),size(W,2) )*min( size(V,1),size(V,2) );
Z_norm_unit = Z_norm;

K_r0= 0.02;
K_r1= 0;
v_r0 = -K_r0*zeta;
v_r1 = -K_r1*(Z_norm+Z_max)*zeta;

v_ad_comp = v_ad + v_r1 +v_r0;


end

== matlab function F16ASYM_Controlled/NDI/NDI: RECONFIG/Pre-Inverter ==
  data: p_dot_comm input; L_comm output; q_dot_comm input; r_dot_comm input; M_comm output; N_comm output; omega_b input
function [L_comm,M_comm,N_comm] = Pre_inverter(p_dot_comm,q_dot_comm,r_dot_comm,omega_b)
Jy  = 75673.6;
Jxz = 1331.4; 
Jz  = 85552.1;  
Jx  = 12874.8;
h_E = 216.9;

Gamma = Jx * Jz - (Jxz  * Jxz);
C1 = ((Jy - Jz)  * Jz  - (Jxz * Jxz))/ Gamma;
C2 = ((Jx - Jy + Jz ) * Jxz ) / Gamma;
C3 = Jz / Gamma;
C4 = Jxz / Gamma;
C5 = (Jz - Jx) / Jy;
C6 = Jxz / Jy ;
C7 = 1 / Jy;
C8 = (Jx * (Jx - Jy ) + Jxz * Jxz) / Gamma;
C9 = Jx / Gamma;



L_comm = -( C4*r_dot_comm+(C2*C9-C4*C8)*omega_b(1)*omega_b(2)+(C2*C4+C1*C9)*omega_b(2)*omega_b(3)-C9*p_dot_comm )/(C3*C9-C4^2);

M_comm = (q_dot_comm-C5*omega_b(1)*omega_b(3)+C6*omega_b(1)^2-C6*omega_b(3)^2 +C7*h_E*omega_b(3))/C7;

N_comm = ( C3*r_dot_comm-C4*p_dot_comm+(C4*C1+C3*C2)*omega_b(2)*omega_b(3)+(C4*C2-C3*C8)*omega_b(1)*omega_b(2)+(C4^2-C3*C9)*h_E*omega_b(2) )/(C3*C9-C4^2);

== matlab function F16ASYM_Controlled/Primary Controller/P controller + adaptive Isolated NN/On-line (adaptive) multi-layer NNs SIMPL/Long Chanel/Long HL NN A_w_z/Long NN ==
  data: X_bar input size=[10,1]; v_ad_comp output; e input; F input; Ks input; B input; Long_learnign_rate input size=1; Long_reg_param input size=1; W input size=[1,31]; V input size=[30,10]; v_ad output; Z_norm_unit output; T_sim parameter; W_update output; V_update output
function [v_ad_comp,v_ad,Z_norm_unit,W_update,V_update]  = Long_AoA_NN(X_bar,e, F, Ks,B,Long_learnign_rate,Long_reg_param,W,V,T_sim)

%% Compute prelimiary parametes Ks(1)=K_b_alpha  and Ks(2) = K_b_q
P = [   1/Ks(1) , F/(Ks(1)^2+Ks(1)*Ks(2));
     1/(Ks(1)^2+Ks(1)*Ks(2)) ,(Ks(1)^2+Ks(1)*Ks(2)+F^2)/(Ks(2)^2*Ks(1)+Ks(2)*Ks(1)^2) ];
zeta= e'*P*B;
s=zeros(30,1);
z=s;
%% Feedforward
z = V*X_bar;
s=sigmoid(V*X_bar);

sigma = [1 ; s ];
% v_ad = W*sigma;

sigma_grad = (sigma.*(ones(size(sigma))-sigma));

%% Compute the gradients or adaptation laws
Gamma_w= Long_learnign_rate; % W learnign rate
Gamma_v= Long_learnign_rate; %V learning rate
lambda = Long_reg_param;

V_dot=zeros(size(V));
W_dot=zeros(size(W'));

W_dot= -Gamma_w*(  (sigma - sigma_grad.*[1;z] ).*zeta  );
W_dot(2:end,1)= W_dot(2:end,1) - Gamma_w*lambda*norm(zeta)*(W(:,2:end))';

M = W'*zeta.*sigma_grad ;
V_dot= -Gamma_v*( M(2:end)*X_bar'  );
V_dot(:,2:end)= V_dot(:,2:end) - Gamma_v*lambda*norm(zeta).*V(:,2:end);


% % % Other way: Based on notes of Andrew NG
% % W_dot=zeros(size(W));
% % delta2=W'*zeta.*sigma_grad;
% % 
% % V_dot = - Gamma_v*( delta2(2:end)*X_bar');
% % V_dot(:,2:end)= V_dot(:,2:end) - Gamma_v*lambda*norm(zeta).*V(:,2:end);
% % 
% % W_dot = - Gamma_w*( zeta*sigma');
% % W_dot(:,2:end)= W_dot(:,2:end) - Gamma_w*lambda*norm(zeta)*(W(:,2:end));
% % 
% % W_dot = W_dot';


%% Adaptation
W_update = W + T_sim*W_dot';
V_update = V + T_sim*V_dot;

%% re-compute v_ad

z = V*X_bar;
s=sigmoid(V*X_bar);

sigma = [1 ; s(:,1) ];
v_ad = W*sigma;

%% Compute v_ad_comp
Z = [ V,zeros(size(V,1),size(W,2));
    zeros(size(W,1),size(V,2)),W];
    
Z_norm = norm(Z,'fro');
Z_max = 2*min(size(W,1),size(W,2) )*min( size(V,1),size(V,2) );
Z_norm_unit = Z_norm/Z_max;

K_r0= 0.1;
K_r1= 0.001;
v_r0 = -K_r0*zeta;
v_r1 = -K_r1*(Z_norm+Z_max)*zeta;

v_ad_comp = v_ad + v_r1 +v_r0;


end

== matlab function F16ASYM_Controlled/Primary Controller/P controller + adaptive Isolated NN/On-line (adaptive) multi-layer NNs SIMPL/Long Chanel/Long HL NN AoA/Long NN ==
  data: X_bar input size=[10,1]; v_ad_comp output; e input; Ks input; B input; Long_learnign_rate input size=1; Long_reg_param input size=1; W input size=[1,31]; V input size=[30,10]; v_ad output; Z_norm_unit output; T_sim parameter; W_update output; V_update output
function [v_ad_comp,v_ad,Z_norm_unit,W_update,V_update]  = Long_AoA_NN(X_bar,e, Ks,B,Long_learnign_rate,Long_reg_param,W,V,T_sim)

%% Compute prelimiary parametes Ks(1)=K_b_alpha  and Ks(2) = K_b_q
P = [   1/Ks(1) , 1/(Ks(1)^2+Ks(1)*Ks(2));
     1/(Ks(1)^2+Ks(1)*Ks(2)) ,(Ks(1)^2+Ks(1)*Ks(2)+1)/(Ks(2)^2*Ks(1)+Ks(2)*Ks(1)^2) ];
zeta= e'*P*B;
s=zeros(30,1);
z=s;
%% Feedforward
z = V*X_bar;
s=sigmoid(V*X_bar);

sigma = [1 ; s ];
% v_ad = W*sigma;

sigma_grad = (sigma.*(ones(size(sigma))-sigma));

%% Compute the gradients or adaptation laws
Gamma_w= Long_learnign_rate; % W learnign rate
Gamma_v= Long_learnign_rate; %V learning rate
lambda = Long_reg_param;

V_dot=zeros(size(V));
W_dot=zeros(size(W'));

W_dot= -Gamma_w*(  (sigma - sigma_grad.*[1;z] ).*zeta  );
W_dot(2:end,1)= W_dot(2:end,1) - Gamma_w*lambda*norm(zeta)*(W(:,2:end))';

M = W'*zeta.*sigma_grad ;
V_dot= -Gamma_v*( M(2:end)*X_bar'  );
V_dot(:,2:end)= V_dot(:,2:end) - Gamma_v*lambda*norm(zeta).*V(:,2:end);


% % % Other way: Based on notes of Andrew NG
% % W_dot=zeros(size(W));
% % delta2=W'*zeta.*sigma_grad;
% % 
% % V_dot = - Gamma_v*( delta2(2:end)*X_bar');
% % V_dot(:,2:end)= V_dot(:,2:end) - Gamma_v*lambda*norm(zeta).*V(:,2:end);
% % 
% % W_dot = - Gamma_w*( zeta*sigma');
% % W_dot(:,2:end)= W_dot(:,2:end) - Gamma_w*lambda*norm(zeta)*(W(:,2:end));
% % 
% % W_dot = W_dot';


%% Adaptation
W_update = W + T_sim*W_dot';
V_update = V + T_sim*V_dot;

%% re-compute v_ad

z = V*X_bar;
s=sigmoid(V*X_bar);

sigma = [1 ; s(:,1) ];
v_ad = W*sigma;

%% Compute v_ad_comp
Z = [ V,zeros(size(V,1),size(W,2));
    zeros(size(W,1),size(V,2)),W];
    
Z_norm = norm(Z,'fro');
Z_max = 2*min(size(W,1),size(W,2) )*min( size(V,1),size(V,2) );
Z_norm_unit = Z_norm;

K_r0= 0.02;
K_r1= 0;
v_r0 = -K_r0*zeta;
v_r1 = -K_r1*(Z_norm+Z_max)*zeta;

v_ad_comp = v_ad + v_r1 +v_r0;


end

== matlab function F16ASYM_Controlled/Primary Controller/P controller + adaptive Isolated NN/On-line (adaptive) multi-layer NNs SIMPL/Roll NN/Roll 1HL NN/Roll NN ==
  data: X_bar input size=[8,1]; v_ad_comp output; e input; P input; B input; Roll_learnign_rate input size=1; Roll_reg_param input size=1; W input size=[1,31]; V input size=[30,8]; v_ad output; Z_norm_unit output; T_sim parameter; W_update output size=[1,31]; V_update output size=[30,8]
function [v_ad_comp,v_ad,Z_norm_unit,W_update,V_update]  = Roll_NN(X_bar,e,P,B,Roll_learnign_rate,Roll_reg_param,W,V,T_sim)

%% Compute prelimiary parametes
zeta= e'*P*B;
s=zeros(30,1);
z=s;
%% Feedforward
z = V*X_bar;
s=sigmoid(V*X_bar);

sigma = [1 ; s ];
% v_ad = W*sigma;

sigma_grad = (sigma.*(ones(size(sigma))-sigma));

%% Compute the gradients or adaptation laws
Gamma_w= Roll_learnign_rate; % W learnign rate
Gamma_v= Roll_learnign_rate; %V learning rate
lambda = Roll_reg_param;

V_dot=zeros(size(V));
W_dot=zeros(size(W'));

W_dot= -Gamma_w*(  (sigma - sigma_grad.*[1;z] ).*zeta  );
W_dot(2:end,1)= W_dot(2:end,1) - Gamma_w*lambda*norm(zeta)*(W(:,2:end))';

M = W'*zeta.*sigma_grad ;
V_dot= -Gamma_v*( M(2:end)*X_bar'  );
V_dot(:,2:end)= V_dot(:,2:end) - Gamma_v*lambda*norm(zeta).*V(:,2:end);


% Other way: Based on notes of Andrew NG
% % % % W_dot=zeros(size(W));
% % % % delta2=W'*zeta.*sigma_grad;
% % % % 
% % % % V_dot = - Gamma_v*( delta2(2:end)*X_bar');
% % % % V_dot(:,2:end)= V_dot(:,2:end) - Gamma_v*lambda*norm(zeta).*V(:,2:end);
% % % % 
% % % % W_dot = - Gamma_w*( zeta*sigma');
% % % % W_dot(:,2:end)= W_dot(:,2:end) - Gamma_w*lambda*norm(zeta)*(W(:,2:end));
% % % % 
% % % % W_dot = W_dot';


%% Adaptation
W_update = W + T_sim*W_dot';
V_update = V + T_sim*V_dot;

%% re-compute v_ad

z = V*X_bar;
s=sigmoid(V*X_bar);

sigma = [1 ; s(:,1) ];
v_ad = W*sigma;

%% Compute v_ad_comp
Z = [ V,zeros(size(V,1),size(W,2));
    zeros(size(W,1),size(V,2)),W];
    
Z_norm = norm(Z,'fro');
Z_max = 2*min(size(W,1),size(W,2) )*min( size(V,1),size(V,2) );
Z_norm_unit = Z_norm;

K_r0= 0;
K_r1= 0;
v_r0 = -K_r0*zeta;
v_r1 = -K_r1*(Z_norm+Z_max)*zeta;
v_ad_comp = v_ad + v_r1 +v_r0;

% % K_r1= 1;
% % v_r1 = - K_r1*(Z_norm+Z_max)*zeta;
% % 
% % v_ad_comp = v_ad + v_r1 ;



end

== matlab function F16ASYM_Controlled/Primary Controller/P controller + adaptive Isolated NN/On-line (adaptive) multi-layer NNs SIMPL/Roll NN/Roll 2HL NN/Roll Multilayer NN ==
  data: X_bar input size=[12,1]; v_ad_comp output; e input size=1; P input; B input; Roll_learnign_rate input size=1; Roll_reg_param input size=1; Theta_1 input size=[30,12]; Theta_2 input size=[20,31]; Theta_3 input size=[1,21]; v_ad output; Z_norm_unit output; T_sim parameter; Theta_1_update output; Theta_2_update output; Theta_3_update output
function [v_ad_comp,v_ad,Z_norm_unit,Theta_1_update,Theta_2_update,Theta_3_update]  = Roll_ML_NN(X_bar,e,P,B,Roll_learnign_rate, Roll_reg_param,Theta_1,Theta_2,Theta_3,T_sim)

%% Compute prelimiary parameters
zeta= e'*P*B;

%% Feedforward. Layers: Sigmoidal, linear, linear

a2=[1 ;  sigmoid( Theta_1*X_bar )]; % Sigmoidal
a3=[1 ;  (Theta_2*a2)]; % Linear
% z4=Theta_3*a3;
% a4 = z4; % Linear
% v_ad =a4;

% Backward
% % delta4=zeta; % In this particular case of adaptive NN, this error is a weighted tracking error
delta3=Theta_3'*zeta;
delta2=Theta_2'*delta3(2:end).*(a2.*(ones(size(a2))-a2)); 


%% Compute the gradients or adaptation laws
Gamma_Theta_3= Roll_learnign_rate; %  learnign rate
Gamma_Theta_2 = Roll_learnign_rate; % learning rate
Gamma_Theta_1= Roll_learnign_rate; % learning rate
lambda = Roll_reg_param;    % Regularization constant

% % Theta_1_dot=zeros(size(Theta_1));
% % Theta_2_dot=zeros(size(Theta_2));
% % Theta_3_dot=zeros(size(Theta_3));

Theta_3_dot = -Gamma_Theta_3*zeta*a3' ;
Theta_3_dot(:,2:end) =  Theta_3_dot(:,2:end) - Gamma_Theta_3*lambda*norm(zeta).*Theta_3(:,2:end);

Theta_2_dot= -Gamma_Theta_2*( delta3(2:end)*a2'   + lambda*norm(zeta).*Theta_2);
Theta_2_dot(:,2:end) =  Theta_2_dot(:,2:end) - Gamma_Theta_2*lambda*norm(zeta).*Theta_2(:,2:end);

Theta_1_dot= -Gamma_Theta_1*( delta2(2:end)*X_bar'   + lambda*norm(zeta).*Theta_1);
Theta_1_dot(:,2:end) =  Theta_1_dot(:,2:end) - Gamma_Theta_1*lambda*norm(zeta).*Theta_1(:,2:end);


%% Adaptation
Theta_1_update = Theta_1 + T_sim*Theta_1_dot;
Theta_2_update = Theta_2 + T_sim*Theta_2_dot;
Theta_3_update = Theta_3 + T_sim*Theta_3_dot;

%% re-compute v_ad

a2=[1 ;  sigmoid( Theta_1_update*X_bar )]; % Sigmoidal
a3=[1 ;  (Theta_2_update*a2)]; % Linear
v_ad=Theta_3_update*a3;


%% Compute v_ad_comp
% Z = blkdiag( Theta_1_update , Theta_2_update , Theta_3_update );

Z =  [ Theta_1_update, zeros(size(Theta_1_update,1),size(Theta_2_update,2)) , zeros(size(Theta_1_update,1),size(Theta_3_update,2));
            zeros(size(Theta_2_update,1),size(Theta_1_update,2)) , Theta_2_update , zeros(size(Theta_2_update,1),size(Theta_3_update,2)) ;
            zeros(size(Theta_3_update,1),size(Theta_1_update,2)),zeros(size(Theta_3_update,1),size(Theta_2_update,2)),  Theta_3_update ];

Z_norm = norm(Z,'fro');
Z_max = min(size(Theta_1))*min(size(Theta_2))*min(size(Theta_3));
Z_norm_unit = Z_norm;

K_r0= 0.02;
K_r1= 0;
v_r0 = -K_r0*zeta;
v_r1 = -K_r1*(Z_norm+Z_max)*zeta;

v_ad_comp = v_ad + v_r1 +v_r0;


end

== matlab function F16ASYM_Controlled/Primary Controller/P controller + adaptive Isolated NN/On-line (adaptive) multi-layer NNs SIMPL/Yaw Chanel/Yaw HL NN/Yaw NN ==
  data: X_bar input size=[12,1]; v_ad_comp output; e input; Ks input; B input; Long_learnign_rate input size=1; Long_reg_param input size=1; W input size=[1,31]; V input size=[30,12]; v_ad output; Z_norm_unit output; T_sim parameter; W_update output; V_update output
function [v_ad_comp,v_ad,Z_norm_unit,W_update,V_update]  = Yaw_NN(X_bar,e, Ks,B,Long_learnign_rate,Long_reg_param,W,V,T_sim)

%% Compute prelimiary parametes Ks(1)=K_b_alpha  and Ks(2) = K_b_q
P = [   1/Ks(1) , 1/(Ks(1)^2+Ks(1)*Ks(2));
     1/(Ks(1)^2+Ks(1)*Ks(2)) ,(Ks(1)^2+Ks(1)*Ks(2)+1)/(Ks(2)^2*Ks(1)+Ks(2)*Ks(1)^2) ];
zeta= e'*P*B;
s=zeros(30,1);
z=s;
%% Feedforward
z = V*X_bar;
s=sigmoid(V*X_bar);

sigma = [1 ; s ];
% v_ad = W*sigma;

sigma_grad = (sigma.*(ones(size(sigma))-sigma));

%% Compute the gradients or adaptation laws
Gamma_w= Long_learnign_rate; % W learnign rate
Gamma_v= Long_learnign_rate; %V learning rate
lambda = Long_reg_param;

V_dot=zeros(size(V));
W_dot=zeros(size(W'));

W_dot= -Gamma_w*(  (sigma - sigma_grad.*[1;z] ).*zeta  );
W_dot(2:end,1)= W_dot(2:end,1) - Gamma_w*lambda*norm(zeta)*(W(:,2:end))';

M = W'*zeta.*sigma_grad ;
V_dot= -Gamma_v*( M(2:end)*X_bar'  );
V_dot(:,2:end)= V_dot(:,2:end) - Gamma_v*lambda*norm(zeta).*V(:,2:end);


% % % Other way: Based on notes of Andrew NG
% % W_dot=zeros(size(W));
% % delta2=W'*zeta.*sigma_grad;
% % 
% % V_dot = - Gamma_v*( delta2(2:end)*X_bar');
% % V_dot(:,2:end)= V_dot(:,2:end) - Gamma_v*lambda*norm(zeta).*V(:,2:end);
% % 
% % W_dot = - Gamma_w*( zeta*sigma');
% % W_dot(:,2:end)= W_dot(:,2:end) - Gamma_w*lambda*norm(zeta)*(W(:,2:end));
% % 
% % W_dot = W_dot';


%% Adaptation
W_update = W + T_sim*W_dot';
V_update = V + T_sim*V_dot;

%% re-compute v_ad

z = V*X_bar;
s=sigmoid(V*X_bar);

sigma = [1 ; s(:,1) ];
v_ad = W*sigma;

%% Compute v_ad_comp
Z = [ V,zeros(size(V,1),size(W,2));
    zeros(size(W,1),size(V,2)),W];
    
Z_norm = norm(Z,'fro');
Z_max = 2*min(size(W,1),size(W,2) )*min( size(V,1),size(V,2) );
Z_norm_unit = Z_norm;

K_r0= 0.02;
K_r1= 0;
v_r0 = -K_r0*zeta;
v_r1 = -K_r1*(Z_norm+Z_max)*zeta;

v_ad_comp = v_ad + v_r1 +v_r0;


end

== matlab function F16ASYM_Controlled/NDI/NDI: NO RECONFIG/Pre-Inverter ==
  data: p_dot_comm input; L_comm output; q_dot_comm input; r_dot_comm input; M_comm output; N_comm output; omega_b input
function [L_comm,M_comm,N_comm] = Pre_inverter(p_dot_comm,q_dot_comm,r_dot_comm,omega_b)
Jy  = 75673.6;
Jxz = 1331.4; 
Jz  = 85552.1;  
Jx  = 12874.8;
h_E = 216.9;

Gamma = Jx * Jz - (Jxz  * Jxz);
C1 = ((Jy - Jz)  * Jz  - (Jxz * Jxz))/ Gamma;
C2 = ((Jx - Jy + Jz ) * Jxz ) / Gamma;
C3 = Jz / Gamma;
C4 = Jxz / Gamma;
C5 = (Jz - Jx) / Jy;
C6 = Jxz / Jy ;
C7 = 1 / Jy;
C8 = (Jx * (Jx - Jy ) + Jxz * Jxz) / Gamma;
C9 = Jx / Gamma;



L_comm = -( C4*r_dot_comm+(C2*C9-C4*C8)*omega_b(1)*omega_b(2)+(C2*C4+C1*C9)*omega_b(2)*omega_b(3)-C9*p_dot_comm )/(C3*C9-C4^2);

M_comm = (q_dot_comm-C5*omega_b(1)*omega_b(3)+C6*omega_b(1)^2-C6*omega_b(3)^2 +C7*h_E*omega_b(3))/C7;

N_comm = ( C3*r_dot_comm-C4*p_dot_comm+(C4*C1+C3*C2)*omega_b(2)*omega_b(3)+(C4*C2-C3*C8)*omega_b(1)*omega_b(2)+(C4^2-C3*C9)*h_E*omega_b(2) )/(C3*C9-C4^2);

== matlab function F16ASYM_Controlled/Control allocator/Control allocator: RECONFIG/MATLAB Function ==
  data: Deflections input; Saturations output; Sup_lim input; Inf_lim input
function Saturations = Saturations(Deflections,Sup_lim,Inf_lim)
Saturations=zeros(7,1);

for i=1:7
    
    if Deflections(i)>=Sup_lim(i)
        Saturations(i)=1;
    elseif Deflections(i)<=Inf_lim(i)
        Saturations(i)=-1;
    else
        Saturations(i)=0;
    end
end

== matlab function F16ASYM_Controlled/Anti-windup Calculation/Anti-windup: Reconfigurable/Ang Accel ==
  data: L input; p_dot output; q_dot output; r_dot output; M input; N input; omega_b input
function [p_dot,q_dot,r_dot] = Ang_accel(L,M,N,omega_b)
Jy  = 75673.6;
Jxz = 1331.4; 
Jz  = 85552.1;  
Jx  = 12874.8;
h_E = 216.9;

denom = Jx*Jz - Jxz*Jxz;

% % C1 = ((Jy - Jz)  * Jz  - (Jxz * Jxz))/ Gamma;
% % C2 = ((Jx - Jy + Jz ) * Jxz ) / Gamma;
% % C3 = Jz / Gamma;
% % C4 = Jxz / Gamma;
% % C5 = (Jz - Jx) / Jy;
% % C6 = Jxz / Jy ;
% % C7 = 1 / Jy;
% % C8 = (Jx * (Jx - Jy ) + Jxz * Jxz) / Gamma;
% % C9 = Jx / Gamma;


p_dot =  (Jz*L + Jxz*N - (Jz*(Jz-Jy)+Jxz*Jxz)*omega_b(2)*omega_b(3) + Jxz*(Jx-Jy+Jz)*omega_b(1)*omega_b(2) + Jxz*omega_b(2)*h_E)/denom;

q_dot = (M + (Jz-Jx)*omega_b(1)*omega_b(3) - Jxz*(omega_b(1)*omega_b(1)-omega_b(3)*omega_b(3)) - omega_b(3)*h_E)/Jy;


r_dot = (Jx*N + Jxz*L + (Jx*(Jx-Jy)+Jxz*Jxz)*omega_b(1)*omega_b(2) - Jxz*(Jx-Jy+Jz)*omega_b(2)*omega_b(3) +  Jx*omega_b(2)*h_E)/denom;

== matlab function F16ASYM_Controlled/Primary Controller/P controller + adaptive Crossed NN/Complete crossed On-line (adaptive) multi-layer NN/Complete crossed On-line (adaptive) multi-layer NN: A_w_z/Cross NN A_w_z ==
  data: X_bar input size=[25,1]; v_ad_comp output; e input; Factor_F input; K_roll input; Ks_long input; Ks_yaw input; B input; Learnign_rate input size=1; Reg_param input size=1; W input size=[3,51]; V input size=[50,25]; v_ad output; Z_norm_unit output; T_sim parameter; W_update output; V_update output
function [v_ad_comp,v_ad,Z_norm_unit,W_update,V_update]  = Cross_NN(X_bar,e,Factor_F, K_roll,Ks_long,Ks_yaw,B,Learnign_rate,Reg_param,W,V,T_sim)

%% Compute prelimiary parametes
% Compute P with regular Lyapunov equation solution
P_roll=1/K_roll;
P_long =  [   1/Ks_long(1) , Factor_F/(Ks_long(1)^2+Ks_long(1)*Ks_long(2));
     1/(Ks_long(1)^2+Ks_long(1)*Ks_long(2)) ,(Ks_long(1)^2+Ks_long(1)*Ks_long(2)+Factor_F^2)/(Ks_long(2)^2*Ks_long(1)+Ks_long(2)*Ks_long(1)^2) ];
P_yaw = [   1/Ks_yaw(1) , 1/(Ks_yaw(1)^2+Ks_yaw(1)*Ks_yaw(2));
     1/(Ks_yaw(1)^2+Ks_yaw(1)*Ks_yaw(2)) ,(Ks_yaw(1)^2+Ks_yaw(1)*Ks_yaw(2)+1)/(Ks_yaw(2)^2*Ks_yaw(1)+Ks_yaw(2)*Ks_yaw(1)^2) ];
 
P = blkdiag(P_roll,P_long,P_yaw);

% % % % Compute P with on-line Lyapunov equation solution
% % % CROSS = 0;
% % % A = [ -K_roll,0,CROSS,0,0;0,-Ks_long(1),1,0,0;
% % %     0,0,-Ks_long(2),0,0;0,0,0,-Ks_yaw(1),Factor_F;0,0,0,0,-Ks_yaw(2)];
% % % 
% % % coder.extrinsic('lyap')
% % % P = A;
% % % P = lyap(A,2*diag(ones(5,1)));



zeta= e'*P*B;

%% Feedforward
z = V*X_bar;
s=sigmoid(V*X_bar);

sigma = [1 ; s ];
% v_ad = W*sigma;

sigma_grad = (sigma.*(ones(size(sigma))-sigma));

%% Compute the gradients or adaptation laws
Gamma_w= Learnign_rate; % W learnign rate
Gamma_v= Learnign_rate; %V learning rate
lambda = Reg_param;

V_dot=zeros(size(V));
W_dot=zeros(size(W));

W_dot= -Gamma_w*(  (sigma - sigma_grad.*[1;z] )*zeta  )';
W_dot(:,2:end)= W_dot(:,2:end) - Gamma_w*lambda*norm(zeta)*(W(:,2:end));

M = W'*zeta'.*sigma_grad ;
V_dot= -Gamma_v*( M(2:end)*X_bar'  );
V_dot(:,2:end)= V_dot(:,2:end) - Gamma_v*lambda*norm(zeta).*V(:,2:end);

% % % % 
% % % % % Other way: Based on notes of Andrew NG
% % % % 
% % % % delta2=W'*zeta'.*sigma_grad;
% % % % 
% % % % V_dot = - Gamma_v*( delta2(2:end)*X_bar');
% % % % V_dot(:,2:end)= V_dot(:,2:end) - Gamma_v*lambda*norm(zeta).*V(:,2:end);
% % % % 
% % % % W_dot = - Gamma_w*( sigma*zeta)';
% % % % W_dot(:,2:end)= W_dot(:,2:end) - Gamma_w*lambda*norm(zeta)*(W(:,2:end));



%% Adaptation
W_update = W + T_sim*W_dot;
V_update = V + T_sim*V_dot;

%% Re-compute v_ad

s=sigmoid(V_update*X_bar);

sigma = [1 ; s(:,1) ];
v_ad = W_update*sigma;

%% Compute v_ad_comp
Z = [ V,zeros(size(V,1),size(W,2));
    zeros(size(W,1),size(V,2)),W];
    
Z_norm = norm(Z,'fro');
Z_max = 2*min(size(W,1),size(W,2) )*min( size(V,1),size(V,2) );
Z_norm_unit = Z_norm;

K_r0= 0.02;
K_r1= 0;
v_r0 = -K_r0*zeta';
v_r1 = -K_r1*(Z_norm+Z_max)*zeta';

v_ad_comp = v_ad + v_r1 +v_r0;


end
